simulink model "Grid Integration till Inverter"  (R2024b)
settings: Solver=VariableStepAuto  StartTime=0.0  StopTime=5  RelTol=1e-3
values from neighbouring files (symbols this model uses):
  Cp_max = 0.48    [parameters.m]
  J = 50    [parameters.m]
  lambda_r = 0.7213    [parameters.m]
  Ld = 0.7029    [parameters.m]
  Lq = 0.7029    [parameters.m]
  P = 8    [parameters.m]
  Rl = 100    [parameters.m]
  Rs = 0.00517    [parameters.m]
  v_cut_in = 0.7    [parameters.m]
libraries: spsDiodeLib x6, spsIGBTLib x6, spsVoltageMeasurementLib x5, simulink x3, spsControlledVoltageSourceLib x3, spsSeriesRLCBranchLib x3, spsGroundLib x2, spsDCVoltageSourceLib x1, spsSawtoothGeneratorLib x1, spsSeriesRLCLoadLib x1, spsThreePhaseParallelRLCBranchLib x1, spsThreePhaseVIMeasurementLib x1
settings Model: Creator=aryan  LastModifiedBy=ASUS

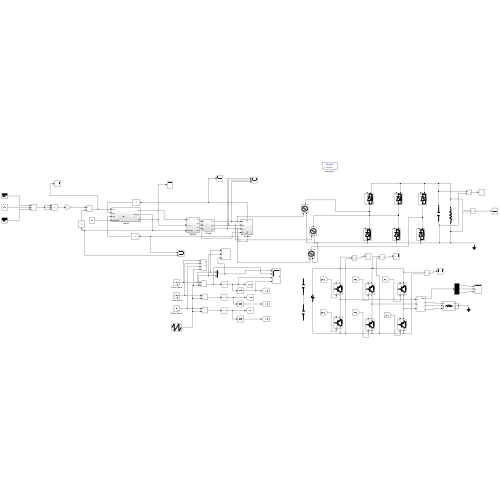
[thumbnail: Simulink's stored preview of the top-level diagram]
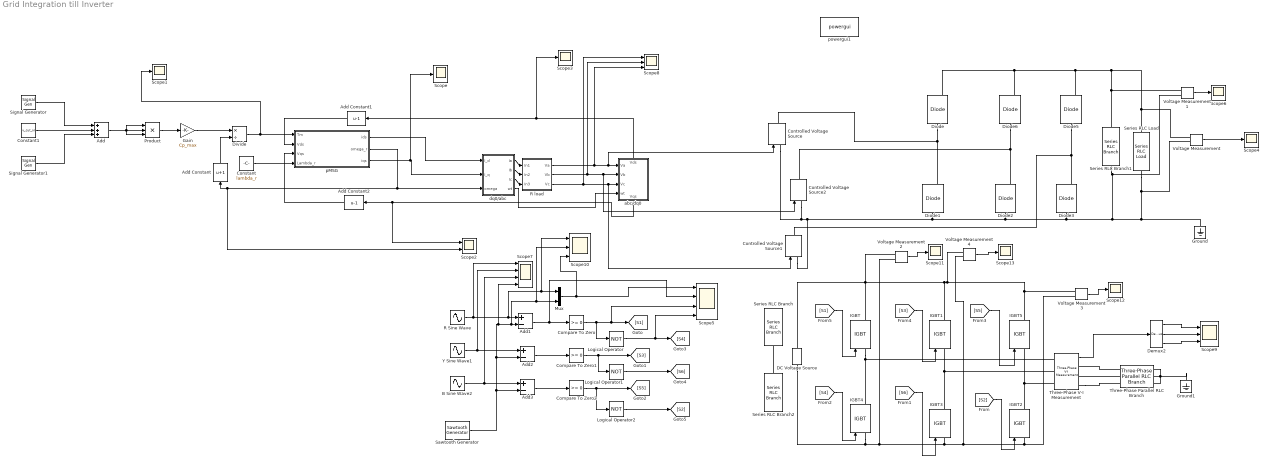
== system Grid Integration till Inverter ==
  Add : Sum  Inputs=+++
  Add Constant : Bias  Bias=1  SaturateOnIntegerOverflow=off
  Add Constant1 : Bias  Bias=-1  SaturateOnIntegerOverflow=off
  Add Constant2 : Bias  Bias=-1  SaturateOnIntegerOverflow=off
  Add1 : Sum  Inputs=+-
  Add2 : Sum  Inputs=+-
  Add3 : Sum  Inputs=+-
  B Sine Wave2 : Sin  Frequency=2*pi*50  Phase=4*pi/3  SampleTime=0
  Compare To Zero : simulink/Logic and Bit Operations/Compare To Zero  relop=>=  OutDataTypeStr=boolean
  Compare To Zero1 : simulink/Logic and Bit Operations/Compare To Zero  relop=>=  OutDataTypeStr=boolean
  Compare To Zero2 : simulink/Logic and Bit Operations/Compare To Zero  relop=>=  OutDataTypeStr=boolean
  Constant : Constant  Value=lambda_r
  Constant1 : Constant  Value=v_cut_in
  Controlled Voltage Source : spsControlledVoltageSourceLib/Controlled Voltage Source  Initialize=on  Source_Type=AC  Amplitude=100  Phase=0  Frequency=60  Measurements=Voltage
  Controlled Voltage Source1 : spsControlledVoltageSourceLib/Controlled Voltage Source  Initialize=on  Source_Type=AC  Amplitude=100  Phase=0  Frequency=60  Measurements=Voltage
  Controlled Voltage Source2 : spsControlledVoltageSourceLib/Controlled Voltage Source  Initialize=on  Source_Type=AC  Amplitude=100  Phase=0  Frequency=60  Measurements=Voltage
  DC Voltage Source : spsDCVoltageSourceLib/DC Voltage Source  Amplitude=400  Measurements=None
  Demux2 : Demux  Outputs=3
  Diode{,1..3,5..6} (6 alike) : spsDiodeLib/Diode  Ron=0.001  Lon=0  Vf=0.8  IC=0  UseSnubber=0  Rs=1000  Cs=1e-9  Measurements=on
  Divide : Product  Inputs=*/
  Gain : Gain  Gain=Cp_max
  Ground : spsGroundLib/Ground  LConnTagsString=a
  Ground1 : spsGroundLib/Ground  LConnTagsString=a
  IGBT{,1..5} (6 alike) : spsIGBTLib/IGBT  Ron=0.001  Lon=0  Vf=1  Tf=1e-6  Tt=2e-6  IC=0  Rs=1e5  Cs=inf  Measurements=on
  Logical Operator : Logic  Operator=NOT  AllPortsSameDT=off  OutDataTypeStr=boolean
  Logical Operator1 : Logic  Operator=NOT  AllPortsSameDT=off  OutDataTypeStr=boolean
  Logical Operator2 : Logic  Operator=NOT  AllPortsSameDT=off  OutDataTypeStr=boolean
  Mux : Mux  Inputs=2
  Product : Product  Inputs=3
  R Sine Wave : Sin  Frequency=2*pi*50  SampleTime=0
  R load : Subsystem
  Sawtooth Generator : spsSawtoothGeneratorLib/Sawtooth Generator  Freq=1000  Phase=180  Ts=0
  Scope{,1,3..4,6,11..13} (8 alike) : Scope
  Scope10 : Scope  NumInputPorts=3
  Scope2 : Scope  NumInputPorts=2
  Scope5 : Scope  NumInputPorts=4
  Scope7 : Scope  NumInputPorts=4
  Scope8 : Scope  NumInputPorts=3
  Scope9 : Scope  NumInputPorts=3
  Series RLC Branch : spsSeriesRLCBranchLib/Series RLC Branch  LConnTagsString=__new0  RConnTagsString=__new0  BranchType=C  Resistance=1  Inductance=1e-3  SetiL0=off  InitialCurrent=0  Capacitance=5  Setx0=off  InitialVoltage=0  Measurements=None
  Series RLC Branch1 : spsSeriesRLCBranchLib/Series RLC Branch  LConnTagsString=__new0  RConnTagsString=__new0  BranchType=C  Resistance=1  Inductance=1e-3  SetiL0=off  InitialCurrent=0  Capacitance=10  Setx0=off  InitialVoltage=0  Measurements=None
  Series RLC Branch2 : spsSeriesRLCBranchLib/Series RLC Branch  LConnTagsString=__new0  RConnTagsString=__new0  BranchType=C  Resistance=1  Inductance=1e-3  SetiL0=off  InitialCurrent=0  Capacitance=5  Setx0=off  InitialVoltage=0  Measurements=None
  Series RLC Load : spsSeriesRLCLoadLib/Series RLC Load  LConnTagsString=a  RConnTagsString=__new0  NominalVoltage=100  NominalFrequency=60  ActivePower=10e3  InductivePower=0  CapacitivePower=0  Setx0=off  InitialVoltage=0  SetiL0=off  InitialCurrent=0  Measurements=None  LoadType=constant Z
  Signal Generator : SignalGenerator  Units=rad/sec
  Signal Generator1 : SignalGenerator  Amplitude=0.5  Frequency=2  Units=rad/sec
  Three-Phase Parallel RLC Branch : spsThreePhaseParallelRLCBranchLib/Three-Phase Parallel RLC Branch  LConnTagsString=A|B|C  RConnTagsString=A|B|C  BranchType=R  Resistance=1  Inductance=1e-3  Capacitance=1e-6  Measurements=None
  Three-Phase V-I Measurement : spsThreePhaseVIMeasurementLib/Three-Phase V-I Measurement  VoltageMeasurement=phase-to-ground  SetLabelV=off  LabelV=Vabc  Vpu=off  VpuLL=off  CurrentMeasurement=no  SetLabelI=off  LabelI=Iabc  Ipu=off  Pbase=100e6  Vbase=500e3  OutputType=Complex  PhasorSimulation=off  PSBequivalent=0
  Voltage Measurement{,1..4} (5 alike) : spsVoltageMeasurementLib/Voltage Measurement  PhasorSimulation=off  OutputType=Complex  PSBequivalent=0
  Y Sine Wave1 : Sin  Frequency=2*pi*50  Phase=2*pi/3  SampleTime=0
  abc/dq0 : Subsystem
      settings: PortSchema="{\"entries\":[{\"content\":{\"sides\":[{\"content\":{\"connectorIds\":[\"In1\",\"In2\",\"In3\",\"In4\"]},\"type\":\"ConnectorPlacement.EquallySpacedRectSide\",\"uuid\":\"2fac6407-f29c-4cbd-80a5-d5c8b501ff3f\"},{\"content\":{\"side\":\"RIGHT\"},\"type\":\"ConnectorPlacement.EquallySpacedRectSide\",\"uuid\":\"b4199395-18e6-46ca-8ed5-7659604401fc\"},{\"content\":{\"connectorIds\":[\"Out2\"],\"side\":\"TOP\"},\"type\":\"ConnectorPlacement.EquallySpacedRectSide\",\"uuid\":\"7e076da1-f59c-4bb1-b41c-85bae00fe7ce\"},{\"content\":{\"connectorIds\":[\"Out1\"],\"side\":\"BOTTOM\"},\"type\":\"ConnectorPlacement.EquallySpacedRectSide\",\"uuid\":\"87f67d1b-7431-4711-8de5-c26f8d6c1f62\"}]},\"type\":\"ConnectorPlacement.EquallySpacedConnector\",\"uuid\":\"270cdb4d-24f2-4849-b248-cc9e04a0d2d1\"}],\"packageUris\":[\"http://schema.mathworks.com/mf0/Connector/R2020b\"],\"version\":\"1.0\"}"
  dq0/abc : Subsystem
  pMSG : Subsystem
  powergui1 : spspowerguiLib/powergui  Priority=1  SimulationMode=Discrete  SampleTime=50e-6  frequency=60  Iterations=50  frequencyindice=0  Pbase=100e6  ErrMax=1e-4  UnitsV=kV  UnitsW=MW  buscounter=0  FunctionMessages=off  echomessages=off  EnableUseOfTLC=off  CurrentSourceSwitches=off  DisableSnubberDevices=off  DisableRonSwitches=off  DisableVfSwitches=off  DisplayEquations=off  AutomaticDiscreteSolvers=off  SolverType=Tustin/Backward Euler (TBE)  Interpol=off  ExternalGateDelay=off  methode=off  Ts=100  x0status=blocks  SPID=on  SwTol=0  HookPort=off  NonlinearTolerance=0  nMaxIteration=15  ContinueOnMaxIteration=off  RestoreLinks=warning  ResistiveCurrentMeasurement=off  Frange=[0:2:500]  Ylog=off  Xlog=on  ShowGrid=off  save=off  variable=ZData  structure=0  ZoomFFT=off  StartTime=0.0  cycles=1  DisplayStyle=1  fundamental=60  FreqAxis=off  MaxFrequency=1000  frequencyindicesteady=1  RmsSteady=1  display=off
  wires:
  Constant/1 -> pMSG/4(Lambda_r)
  Divide/1 -> Scope1/1, pMSG/1(Tm)
  pMSG/1(ids) -> dq0/abc/1(I_d)
  dq0/abc/2(Ib) -> R load/2(In2)
  dq0/abc/1(Ia) -> R load/1(In1)
  dq0/abc/4(wt) -> abc/dq0/4(wt)
  dq0/abc/3(Ic) -> R load/3(In3)
  pMSG/3(iqs) -> Scope/1, dq0/abc/2(I_q)
  Add Constant/1 -> Divide/2
  Add/1 -> Product/3, Product/1, Product/2
  Product/1 -> Gain/1
  Gain/1 -> Divide/1
  Add Constant1/1 -> pMSG/2(Vds)
  abc/dq0/2(Vds) -> Scope3/1, Add Constant1/1
  Add Constant2/1 -> pMSG/3(Vqs)
  Signal Generator/1 -> Add/1
  Signal Generator1/1 -> Add/3
  Constant1/1 -> Add/2
  abc/dq0/1(Vqs) -> Scope2/1, Add Constant2/1
  pMSG/2(omega_r) -> Scope2/2, Add Constant/1, dq0/abc/3(omega)
  R load/1(Va) -> Controlled Voltage Source/1, abc/dq0/1(Va), Scope8/3
  Voltage Measurement/1 -> Scope4/1
  R load/3(Vc) -> Scope8/1, Controlled Voltage Source1/1, abc/dq0/3(Vc)
  R load/2(Vb) -> Scope8/2, Controlled Voltage Source2/1, abc/dq0/2(Vb)
  Voltage Measurement1/1 -> Scope6/1
  Y Sine Wave1/1 -> Scope7/2, Add2/1
  B Sine Wave2/1 -> Scope7/3, Add3/1
  Sawtooth Generator/1 -> Add3/2, Add2/2, Scope7/4, Scope10/2, Mux/2, Add1/2
  Add1/1 -> Scope5/2, Compare To Zero/1
  Add2/1 -> Compare To Zero1/1
  Add3/1 -> Compare To Zero2/1
  Compare To Zero/1 -> Logical Operator/1, Scope5/3, [S1]
  Compare To Zero2/1 -> Logical Operator2/1, [S5]
  Compare To Zero1/1 -> Logical Operator1/1, [S3]
  Logical Operator/1 -> Scope5/4, [S4]
  Logical Operator1/1 -> [S6]
  Logical Operator2/1 -> [S2]
  [S1] -> IGBT/1
  [S3] -> IGBT1/1
  [S5] -> IGBT5/1
  [S4] -> IGBT4/1
  [S6] -> IGBT3/1
  [S2] -> IGBT2/1
  Three-Phase V-I Measurement/1 -> Demux2/1
  Demux2/1 -> Scope9/1
  Demux2/2 -> Scope9/2
  Demux2/3 -> Scope9/3
  R Sine Wave/1 -> Scope7/1, Scope10/1, Mux/1, Add1/1
  Mux/1 -> Scope10/3, Scope5/1
  Voltage Measurement2/1 -> Scope11/1
  Voltage Measurement3/1 -> Scope12/1
  Voltage Measurement4/1 -> Scope13/1
  connections:
  Diode/RConn1 -- Diode6/RConn1 -- Diode5/RConn1 -- Series RLC Load/LConn1 -- Voltage Measurement/LConn1 -- Series RLC Branch1/LConn1 -- Voltage Measurement1/LConn1
  Diode/LConn1 -- Controlled Voltage Source/RConn1 -- Diode1/RConn1
  Diode6/LConn1 -- Controlled Voltage Source2/RConn1 -- Diode2/RConn1
  Diode5/LConn1 -- Controlled Voltage Source1/RConn1 -- Diode3/RConn1
  Voltage Measurement1/LConn2 -- Series RLC Branch1/RConn1 -- Diode1/LConn1 -- Controlled Voltage Source1/LConn1 -- Controlled Voltage Source2/LConn1 -- Controlled Voltage Source/LConn1 -- Diode2/LConn1 -- Diode3/LConn1 -- Ground/LConn1 -- Series RLC Load/RConn1 -- Voltage Measurement/LConn2
  IGBT/LConn1 -- IGBT4/RConn1 -- Three-Phase V-I Measurement/LConn1
  IGBT3/RConn1 -- Three-Phase V-I Measurement/LConn2 -- IGBT1/LConn1
  IGBT2/RConn1 -- Three-Phase V-I Measurement/LConn3 -- IGBT5/LConn1
  Three-Phase Parallel RLC Branch/LConn1 -- Three-Phase V-I Measurement/RConn1
  Three-Phase Parallel RLC Branch/LConn2 -- Three-Phase V-I Measurement/RConn2
  Three-Phase V-I Measurement/RConn3 -- Three-Phase Parallel RLC Branch/LConn3
  Three-Phase Parallel RLC Branch/RConn1 -- Ground1/LConn1 -- Three-Phase Parallel RLC Branch/RConn2 -- Three-Phase Parallel RLC Branch/RConn3
  Series RLC Branch2/LConn1 -- Series RLC Branch/RConn1
  Voltage Measurement4/LConn1 -- IGBT5/RConn1 -- Voltage Measurement3/LConn1 -- DC Voltage Source/RConn1 -- IGBT/RConn1 -- Voltage Measurement2/LConn1 -- IGBT1/RConn1
  Voltage Measurement4/LConn2 -- IGBT4/LConn1 -- DC Voltage Source/LConn1 -- Voltage Measurement2/LConn2 -- IGBT3/LConn1 -- IGBT2/LConn1 -- Voltage Measurement3/LConn2

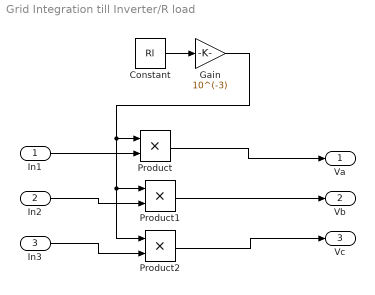
== system Grid Integration till Inverter/R load ==
  In1 : Inport
  In2 : Inport  Port=2
  In3 : Inport  Port=3
  Constant : Constant  Value=Rl
  Gain : Gain  Gain=10^(-3)
  Product : Product
  Product1 : Product
  Product2 : Product
  Va : Outport
  Vb : Outport  Port=2
  Vc : Outport  Port=3
  wires:
  Product/1 -> Va/1
  Product1/1 -> Vb/1
  In1/1 -> Product/2
  In3/1 -> Product2/2
  In2/1 -> Product1/2
  Product2/1 -> Vc/1
  Gain/1 -> Product2/1, Product1/1, Product/1
  Constant/1 -> Gain/1

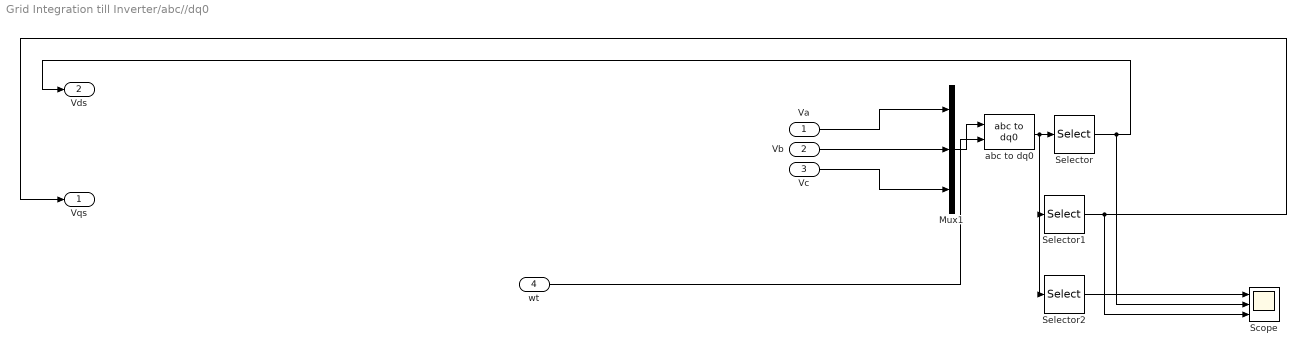
== system Grid Integration till Inverter/abc//dq0 ==
  Va : Inport
  Vb : Inport  Port=2
  Vc : Inport  Port=3
  wt : Inport  Port=4
  Mux1 : Mux  Inputs=3
  Scope : Scope  NumInputPorts=3
  Selector : Selector  InputPortWidth=3  IndexOptions=Index vector (dialog)  Indices=1  OutputSizes=1
  Selector1 : Selector  InputPortWidth=3  IndexOptions=Index vector (dialog)  Indices=2  OutputSizes=1
  Selector2 : Selector  InputPortWidth=3  IndexOptions=Index vector (dialog)  Indices=3  OutputSizes=1
  abc to dq0 : spsabctodq0Lib/abc to dq0  Alignment=90 degrees behind phase A axis
  Vqs : Outport
  Vds : Outport  Port=2
  wires:
  Mux1/1 -> abc to dq0/1
  Vc/1 -> Mux1/3
  wt/1 -> abc to dq0/2
  abc to dq0/1 -> Selector2/1, Selector1/1, Selector/1
  Vb/1 -> Mux1/2
  Va/1 -> Mux1/1
  Selector/1 -> Scope/2, Vds/1
  Selector1/1 -> Scope/3, Vqs/1
  Selector2/1 -> Scope/1

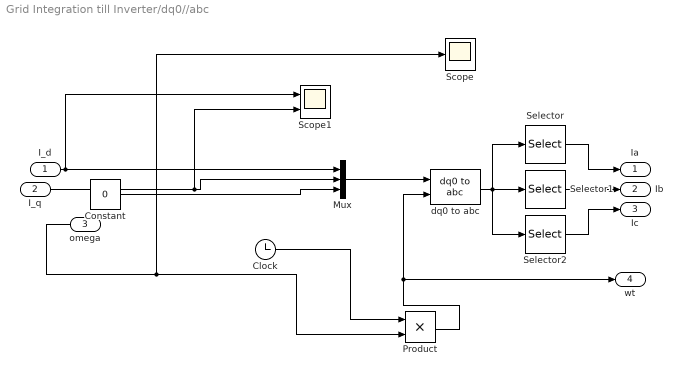
== system Grid Integration till Inverter/dq0//abc ==
  I_d : Inport
  I_q : Inport  Port=2
  omega : Inport  Port=3
  Clock : Clock
  Constant : Constant  Value=0
  Mux : Mux  Inputs=3
  Product : Product
  Scope : Scope
  Scope1 : Scope  NumInputPorts=2
  Selector : Selector  InputPortWidth=3  IndexOptions=Index vector (dialog)  Indices=1  OutputSizes=1
  Selector1 : Selector  InputPortWidth=3  IndexOptions=Index vector (dialog)  Indices=2  OutputSizes=1
  Selector2 : Selector  InputPortWidth=3  IndexOptions=Index vector (dialog)  Indices=3  OutputSizes=1
  dq0 to abc : spsdq0toabcLib/dq0 to abc  Alignment=90 degrees behind phase A axis
  Ia : Outport
  Ib : Outport  Port=2
  Ic : Outport  Port=3
  wt : Outport  Port=4
  wires:
  omega/1 -> Scope/1, Product/2
  Mux/1 -> dq0 to abc/1
  Product/1 -> dq0 to abc/2, wt/1
  Selector2/1 -> Ic/1
  Selector/1 -> Ia/1
  dq0 to abc/1 -> Selector/1, Selector2/1, Selector1/1
  Selector1/1 -> Ib/1
  I_q/1 -> Scope1/2, Mux/2
  Constant/1 -> Mux/3
  Clock/1 -> Product/1
  I_d/1 -> Scope1/1, Mux/1

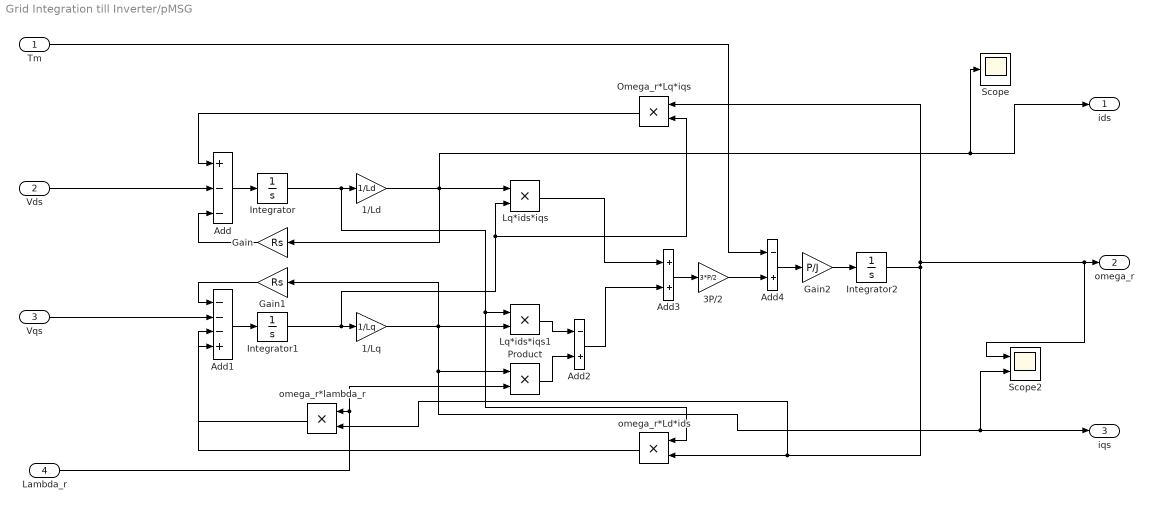
== system Grid Integration till Inverter/pMSG ==
  Tm : Inport
  Vds : Inport  Port=2
  Vqs : Inport  Port=3
  Lambda_r : Inport  Port=4
  1/Ld : Gain  Gain=1/Ld
  1/Lq : Gain  Gain=1/Lq
  3P/2 : Gain  Gain=3*P/2
  Add : Sum  Inputs=+--
  Add1 : Sum  Inputs=---+
  Add2 : Sum  Inputs=-+
  Add3 : Sum
  Add4 : Sum  Inputs=-+
  Gain : Gain  Gain=Rs
  Gain1 : Gain  Gain=Rs
  Gain2 : Gain  Gain=P/J
  Integrator : Integrator
  Integrator1 : Integrator
  Integrator2 : Integrator
  Lq*ids*iqs : Product
  Lq*ids*iqs1 : Product
  Omega_r*Lq*iqs : Product
  Product : Product
  Scope : Scope
  Scope2 : Scope  NumInputPorts=2
  omega_r*Ld*ids : Product
  omega_r*lambda_r : Product
  ids : Outport
  omega_r : Outport  Port=2
  iqs : Outport  Port=3
  wires:
  Lq*ids*iqs/1 -> Add3/1
  Integrator/1 -> omega_r*Ld*ids/1, Lq*ids*iqs1/1, 1/Ld/1
  1/Lq/1 -> Scope2/2, iqs/1, Product/1, Gain1/1, Lq*ids*iqs1/2
  Add4/1 -> Gain2/1
  Omega_r*Lq*iqs/1 -> Add/1
  Add3/1 -> 3P/2/1
  omega_r*lambda_r/1 -> Add1/4
  Gain/1 -> Add/3
  Integrator1/1 -> Omega_r*Lq*iqs/2, Lq*ids*iqs/2, 1/Lq/1
  Tm/1 -> Add4/1
  Lq*ids*iqs1/1 -> Add2/1
  Gain2/1 -> Integrator2/1
  Lambda_r/1 -> omega_r*lambda_r/1, Product/2
  Vds/1 -> Add/2
  Add1/1 -> Integrator1/1
  Product/1 -> Add2/2
  1/Ld/1 -> Scope/1, ids/1, Gain/1, Lq*ids*iqs/1
  Gain1/1 -> Add1/1
  Add/1 -> Integrator/1
  Add2/1 -> Add3/2
  3P/2/1 -> Add4/2
  Vqs/1 -> Add1/2
  omega_r*Ld*ids/1 -> Add1/3
  Integrator2/1 -> omega_r*lambda_r/2, omega_r*Ld*ids/2, Scope2/1, omega_r/1, Omega_r*Lq*iqs/1
